simulink library "aeb"  (Simulink 8.1)
settings: Solver=ode1  StartTime=0.0  StopTime=Inf  FixedStep=0.001  RelTol=1e-3
PostLoadFcn:
  | , if any(exist('dsrtsu_mdlpostloadfcn', 'file') == [2, 3, 6]), try dsrtsu_mdlpostloadfcn('Execute', bdroot); catch fprintf('Error in PostLoadFcn (dsrtsu_mdlpostloadfcn) for model "%s":\n %s\n', bdroot, lasterr); end, end,
undefined symbols (not defined in the file or in its folder): KAEB_AEBAutoBrakeDecelReq_mps2
libraries: seb x1, beb x1
settings Model: DSRTSU_INTERNAL_RTI_VER=450  DSRTSU_INTERNAL_RTI_TYPE=rti1401  RTICANMMDATA=struct('GeneralSetupData',struct('modelroot','D:\ELN150201_TAIWAN\trunk\AdasDragon\software\sw_development\arch\app\aeb','generalsettings',struct('filesettings',struct('destfolder',struct('Name','RTICANMM_FILES','Check',1),'buildfolder',struct('Name','.','Check',1),'AbsDestfolder',struct('Name','D:\ELN150201_TAIWAN\trunk\AdasDragon\software\sw_development\arch\app\aeb\RTICANMM_FILES'),'AbsBuildfolder',struct('Name','D:\ELN150201_TAIWAN\trunk\AdasDragon\software\sw_development\arch\app\aeb'))),'options',struct('addpaths',1,'rmpaths',1,'addtrcexclusion',logical(1),'cannavigator',struct('checkmonitoring',0),'show_usrtrc',0,'use_usrtrc',0),'advanced',struct('options',[1 1 1 1 1 1 1 1 1 1 1 1 1 1 1 1 1 1 1 1 1 1 1 1 1 1 1 1 1 1 1 1 1 1 1 1 1 1 1 1 1 1 1 1 1 1 1 1 1 1 1 1 1 1 1 1 1 1 1 1 1 1 1 1 1 1 1 1 1 1 1 1 1 1 1 1 1 1 1 1 1 1 1 1 1 1 1 1 1 1 1 1 1 1 1 1 1 1 1 1]),'MPSetup',{{}},'modelname','aeb','block','aeb'))  DSRTSU_INTERNAL_RTIFPGA=40  Creator=tescamilla  LastModifiedBy=AT015555

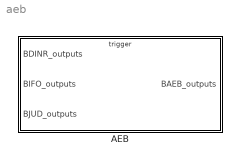
== system aeb ==
  AEB : Subsystem  TreatAsAtomicUnit=on

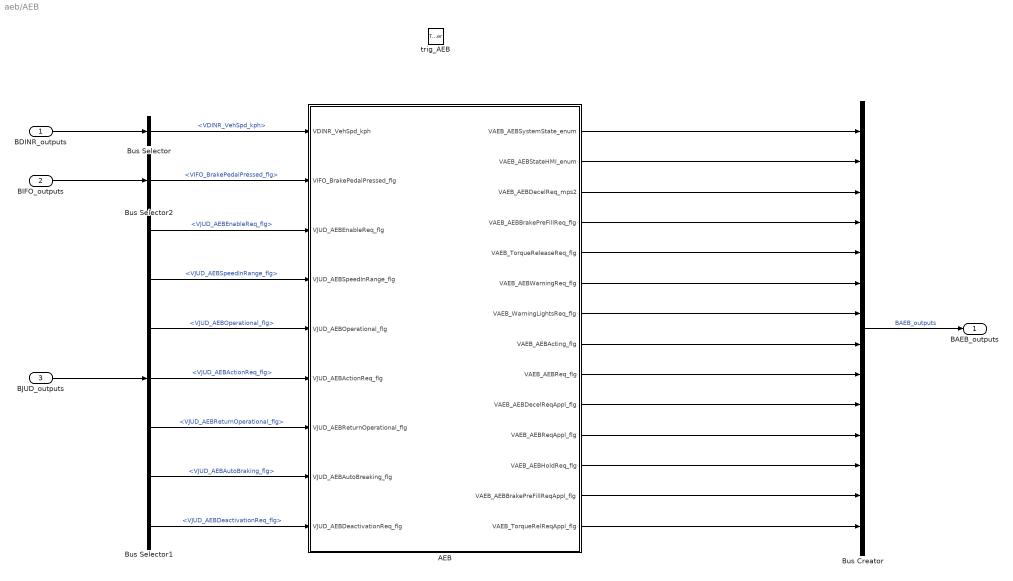
== system aeb/AEB ==
  BDINR_outputs : Inport  OutDataTypeStr=Bus: BDINR_outputs
  BIFO_outputs : Inport  Port=2  OutDataTypeStr=Bus: BIFO_outputs
  BJUD_outputs : Inport  Port=3  OutDataTypeStr=Bus: BJUD_outputs
  trig_AEB : TriggerPort  TriggerType=function-call
      settings: AttributesFormatString=State = %<StatesWhenEnabling>
  AEB : Subsystem
  Bus Creator : BusCreator  Inputs=14  OutDataTypeStr=Bus: BAEB_outputs
  Bus Selector : BusSelector  OutputSignals=VDINR_VehSpd_kph
  Bus Selector1 : BusSelector  OutputSignals=VJUD_AEBEnableReq_flg,VJUD_AEBSpeedInRange_flg,VJUD_AEBOperational_flg,VJUD_AEBActionReq_flg,VJUD_AEBReturnOperational_flg,VJUD_AEBAutoBraking_flg,VJUD_AEBDeactivationReq_flg
  Bus Selector2 : BusSelector  OutputSignals=VIFO_BrakePedalPressed_flg
  BAEB_outputs : Outport  OutDataTypeStr=Bus: BAEB_outputs
  wires:
  BDINR_outputs/1 -> Bus Selector/1
  BJUD_outputs/1 -> Bus Selector1/1
  Bus Selector/1 -> AEB/1(VDINR_VehSpd_kph)  "<VDINR_VehSpd_kph>"
  Bus Creator/1 -> BAEB_outputs/1  "BAEB_outputs"
  BIFO_outputs/1 -> Bus Selector2/1
  Bus Selector2/1 -> AEB/2(VIFO_BrakePedalPressed_flg)  "<VIFO_BrakePedalPressed_flg>"
  Bus Selector1/2 -> AEB/4(VJUD_AEBSpeedInRange_flg)  "<VJUD_AEBSpeedInRange_flg>"
  Bus Selector1/4 -> AEB/6(VJUD_AEBActionReq_flg)  "<VJUD_AEBActionReq_flg>"
  Bus Selector1/3 -> AEB/5(VJUD_AEBOperational_flg)  "<VJUD_AEBOperational_flg>"
  Bus Selector1/6 -> AEB/8(VJUD_AEBAutoBreaking_flg)  "<VJUD_AEBAutoBraking_flg>"
  Bus Selector1/1 -> AEB/3(VJUD_AEBEnableReq_flg)  "<VJUD_AEBEnableReq_flg>"
  Bus Selector1/7 -> AEB/9(VJUD_AEBDeactivationReq_flg)  "<VJUD_AEBDeactivationReq_flg>"
  AEB/2(VAEB_AEBStateHMI_enum) -> Bus Creator/2
  AEB/1(VAEB_AEBSystemState_enum) -> Bus Creator/1
  AEB/4(VAEB_AEBBrakePreFillReq_flg) -> Bus Creator/4
  AEB/5(VAEB_TorqueReleaseReq_flg) -> Bus Creator/5
  AEB/6(VAEB_AEBWarningReq_flg) -> Bus Creator/6
  AEB/8(VAEB_AEBActing_flg) -> Bus Creator/8
  AEB/7(VAEB_WarningLightsReq_flg) -> Bus Creator/7
  AEB/3(VAEB_AEBDecelReq_mps2) -> Bus Creator/3
  AEB/9(VAEB_AEBReq_flg) -> Bus Creator/9
  AEB/10(VAEB_AEBDecelReqAppl_flg) -> Bus Creator/10
  AEB/11(VAEB_AEBReqAppl_flg) -> Bus Creator/11
  AEB/12(VAEB_AEBHoldReq_flg) -> Bus Creator/12
  AEB/13(VAEB_AEBBrakePreFillReqAppl_flg) -> Bus Creator/13
  AEB/14(VAEB_TorqueRelReqAppl_flg) -> Bus Creator/14
  Bus Selector1/5 -> AEB/7(VJUD_AEBReturnOperational_flg)  "<VJUD_AEBReturnOperational_flg>"

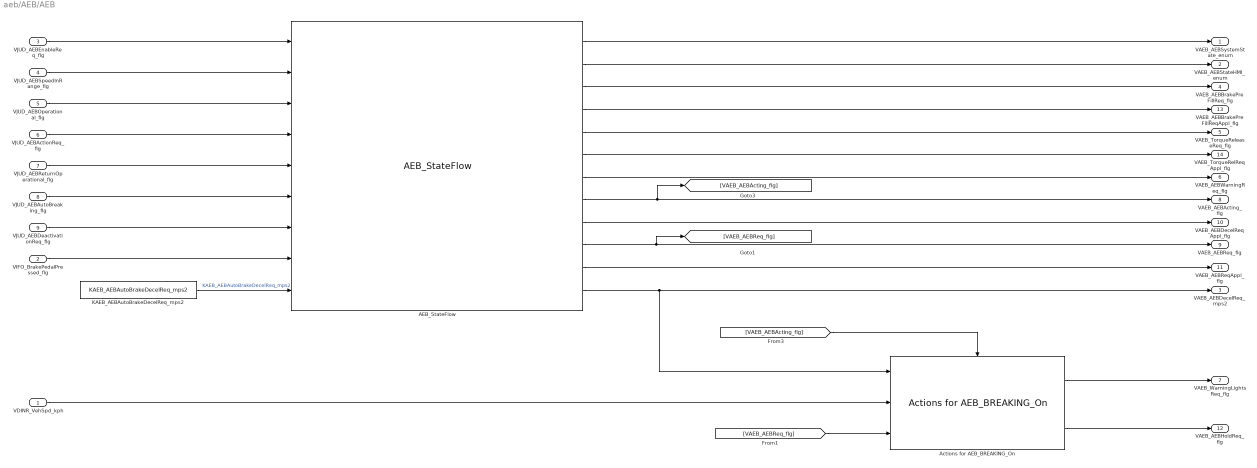
== system aeb/AEB/AEB ==
  VDINR_VehSpd_kph : Inport
  VIFO_BrakePedalPressed_flg : Inport  Port=2
  VJUD_AEBEnableReq_flg : Inport  Port=3
  VJUD_AEBSpeedInRange_flg : Inport  Port=4
  VJUD_AEBOperational_flg : Inport  Port=5
  VJUD_AEBActionReq_flg : Inport  Port=6
  VJUD_AEBReturnOperational_flg : Inport  Port=7
  VJUD_AEBAutoBreaking_flg : Inport  Port=8
  VJUD_AEBDeactivationReq_flg : Inport  Port=9
  AEB_StateFlow : seb/AEB_StateFlow
  Actions for AEB_BREAKING_On : beb/Actions for AEB_BREAKING_On
  KAEB_AEBAutoBrakeDecelReq_mps2 : Constant  Value=KAEB_AEBAutoBrakeDecelReq_mps2
  VAEB_AEBSystemState_enum : Outport  OutDataTypeStr=uint8
  VAEB_AEBStateHMI_enum : Outport  Port=2  OutDataTypeStr=uint8
  VAEB_AEBDecelReq_mps2 : Outport  Port=3  OutDataTypeStr=single
  VAEB_AEBBrakePreFillReq_flg : Outport  Port=4  OutDataTypeStr=boolean
  VAEB_TorqueReleaseReq_flg : Outport  Port=5  OutDataTypeStr=boolean
  VAEB_AEBWarningReq_flg : Outport  Port=6  OutDataTypeStr=boolean
  VAEB_WarningLightsReq_flg : Outport  Port=7  OutDataTypeStr=boolean
  VAEB_AEBActing_flg : Outport  Port=8  OutDataTypeStr=boolean
  VAEB_AEBReq_flg : Outport  Port=9  OutDataTypeStr=boolean
  VAEB_AEBDecelReqAppl_flg : Outport  Port=10  OutDataTypeStr=boolean
  VAEB_AEBReqAppl_flg : Outport  Port=11  OutDataTypeStr=boolean
  VAEB_AEBHoldReq_flg : Outport  Port=12  OutDataTypeStr=boolean
  VAEB_AEBBrakePreFillReqAppl_flg : Outport  Port=13  OutDataTypeStr=boolean
  VAEB_TorqueRelReqAppl_flg : Outport  Port=14  OutDataTypeStr=boolean
  wires:
  Actions for AEB_BREAKING_On/1 -> VAEB_WarningLightsReq_flg/1
  Actions for AEB_BREAKING_On/2 -> VAEB_AEBHoldReq_flg/1
  AEB_StateFlow/2 -> VAEB_AEBStateHMI_enum/1
  AEB_StateFlow/3 -> VAEB_AEBBrakePreFillReq_flg/1
  AEB_StateFlow/5 -> VAEB_TorqueReleaseReq_flg/1
  AEB_StateFlow/1 -> VAEB_AEBSystemState_enum/1
  AEB_StateFlow/7 -> VAEB_AEBWarningReq_flg/1
  VJUD_AEBAutoBreaking_flg/1 -> AEB_StateFlow/6
  VJUD_AEBSpeedInRange_flg/1 -> AEB_StateFlow/2
  VJUD_AEBEnableReq_flg/1 -> AEB_StateFlow/1
  VJUD_AEBActionReq_flg/1 -> AEB_StateFlow/4
  VJUD_AEBDeactivationReq_flg/1 -> AEB_StateFlow/7
  VJUD_AEBOperational_flg/1 -> AEB_StateFlow/3
  AEB_StateFlow/8 -> [VAEB_AEBActing_flg], VAEB_AEBActing_flg/1
  VDINR_VehSpd_kph/1 -> Actions for AEB_BREAKING_On/2
  VIFO_BrakePedalPressed_flg/1 -> AEB_StateFlow/8
  AEB_StateFlow/9 -> VAEB_AEBDecelReqAppl_flg/1
  AEB_StateFlow/11 -> VAEB_AEBReqAppl_flg/1
  AEB_StateFlow/12 -> VAEB_AEBDecelReq_mps2/1, Actions for AEB_BREAKING_On/1
  [VAEB_AEBReq_flg] -> Actions for AEB_BREAKING_On/3
  AEB_StateFlow/10 -> [VAEB_AEBReq_flg], VAEB_AEBReq_flg/1
  AEB_StateFlow/4 -> VAEB_AEBBrakePreFillReqAppl_flg/1
  [VAEB_AEBActing_flg] -> Actions for AEB_BREAKING_On/Enable
  AEB_StateFlow/6 -> VAEB_TorqueRelReqAppl_flg/1
  VJUD_AEBReturnOperational_flg/1 -> AEB_StateFlow/5
  KAEB_AEBAutoBrakeDecelReq_mps2/1 -> AEB_StateFlow/9  "KAEB_AEBAutoBrakeDecelReq_mps2"
